simulink model "Modulated TDPC Q4"  (R2021b)
settings: Solver=ode4  StartTime=0.0  StopTime=20  FixedStep=0.0001  RelTol=1e-3
libraries: slpidlib x2
settings Model: Creator=rmkna  LastModifiedBy=rmkna

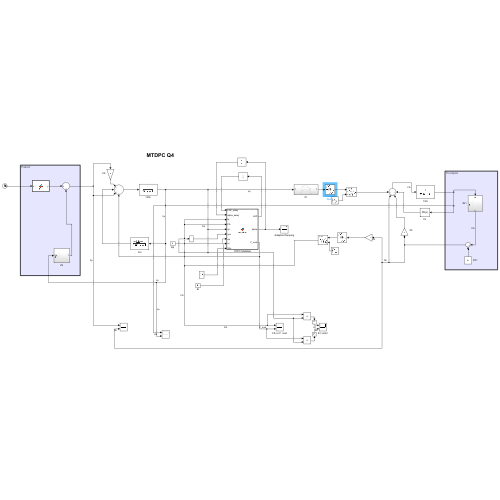
[thumbnail: Simulink's stored preview of the top-level diagram]
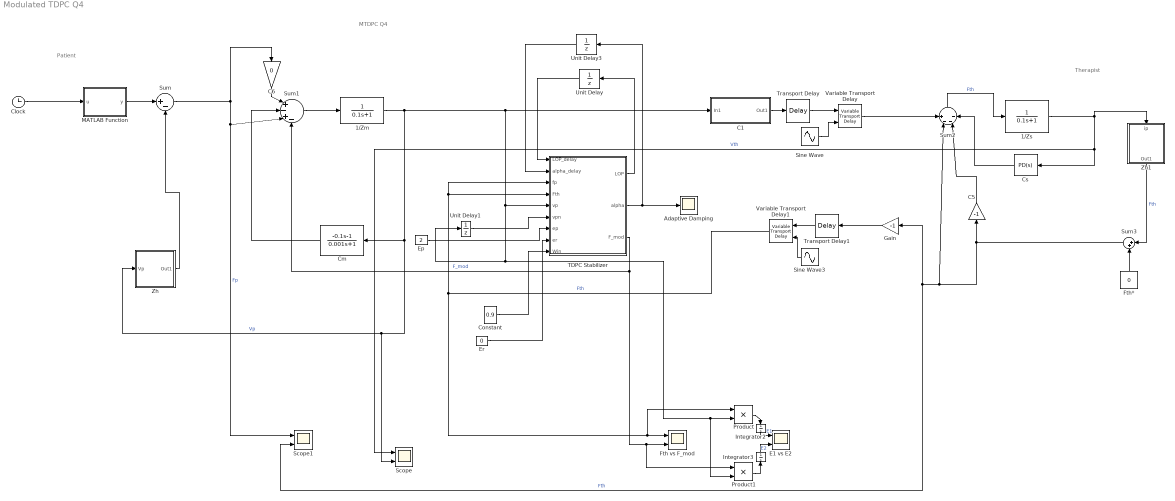
== system Modulated TDPC Q4 ==
  note: MTDPC Q4
  note: Therapist
  note: Patient
  " TDPC Stabilizer" : MATLAB Function  TreatAsAtomicUnit=on
  1/Zm : TransferFcn  Denominator=[0.1 1]
  1/Zs : TransferFcn  Denominator=[0.1 1]
  Adaptive Damping : Scope
  C1 : Subsystem
  "C5 " : Gain  Gain=-1
  "C6 " : Gain  Gain=0
  Clock : Clock
  Cm : TransferFcn  Numerator=[-0.1 -1]  Denominator=[0.001 1]
  Constant : Constant  Value=0.9
  Cs : slpidlib/PID Controller  Controller=PD  Form=Parallel  TimeDomain=Continuous-time  UseExternalTs=off  SampleTime=-1  IntegratorMethod=Forward Euler  FilterMethod=Forward Euler  ControllerParametersSource=internal  P=1000  I=1  D=1  UseFilter=on  N=1000  TunerSelectOption=Transfer Function Based (PID Tuner App)  InitialConditionSource=internal  InitialConditionForIntegrator=0  InitialConditionForFilter=0  DifferentiatorICPrevScaledInput=0  ExternalReset=none  TrackingMode=off  Kt=1  LimitOutput=off  SatLimitsSource=internal  UpperSaturationLimit=inf  LowerSaturationLimit=-inf  LinearizeAsGain=on  AntiWindupMode=none  Kb=1  POutMin=[]  POutMax=[]  IOutMin=[]  IOutMax=[]  DOutMin=[]  DOutMax=[]  NOutMin=[]  NOutMax=[]  SumOutMin=[]  SumOutMax=[]  SaturationOutMin=[]  SaturationOutMax=[]  PParamMin=[]  PParamMax=[]  IParamMin=[]  IParamMax=[]  DParamMin=[]  DParamMax=[]  NParamMin=[]  NParamMax=[]  KbParamMin=[]  KbParamMax=[]  KtParamMin=[]  KtParamMax=[]  KbOutMin=[]  KbOutMax=[]  KtOutMin=[]  KtOutMax=[]  IntegratorOutMin=[]  IntegratorOutMax=[]  FilterOutMin=[]  FilterOutMax=[]  SumI1OutMin=[]  SumI1OutMax=[]  SumI2OutMin=[]  SumI2OutMax=[]  SumI3OutMin=[]  SumI3OutMax=[]  SumI4OutMin=[]  SumI4OutMax=[]  SumDOutMin=[]  SumDOutMax=[]  DifferentiatorOutMin=[]  DifferentiatorOutMax=[]  FilterDiffOutCoefMin=[]  FilterDiffOutCoefMax=[]  ReciprocalOutMin=[]  ReciprocalOutMax=[]  SumDenOutMin=[]  SumDenOutMax=[]  SumNumOutMin=[]  SumNumOutMax=[]  DivideOutMin=[]  DivideOutMax=[]  UdiffTsProdOutMin=[]  UdiffTsProdOutMax=[]  NTsProdOutMin=[]  NTsProdOutMax=[]  UintegralTsProdOutMin=[]  UintegralTsProdOutMax=[]  UngainTsProdOutMin=[]  UngainTsProdOutMax=[]  IntegratorContinuousStateAttributes=''  IntegratorStateMustResolveToSignalObject=off  IntegratorRTWStateStorageClass=Auto  FilterContinuousStateAttributes=''  FilterStateMustResolveToSignalObject=off  FilterRTWStateStorageClass=Auto  ParallelPVariant=InternalParameters  IdealPVariant=Disabled  IVariant=Disabled  DVariant=InternalParameters  IntegratorVariant=Disabled  SatVariant=Disabled  AWVariant=Disabled  PCopyVariant=Disabled  TRVariant=Disabled  FdbkBlocksVariant=Forward  IdealPFdbkVariant=Disabled  SatFdbkVariant=Disabled  DerivativeFilterVariant=ContFilter  NVariant=InternalParameters  NCopyVariant=Disabled  FilterICVariant=InternalICsFilter  IntegratorICVariant=Disabled  ExternalResetVariant=Disabled  TRSumVariant=Passthrough  SumFdbkVariant=Disabled  SumVariant=Sum_PD  TsampFilterVariant=InternalTs  TsampNgainVariant=Passthrough  TsampIntegralVariant=Disabled_SignalSpec  ExternalSaturationOutDataTypeStr=Inherit: Same as second input
  E1 vs E2 : Scope  NumInputPorts=2
  Ep : Constant  Value=2
  Er : Constant  Value=0
  Fth vs F_mod : Scope  NumInputPorts=2
  Fth* : Constant  Value=0  OutDataTypeStr=Inherit: Inherit via back propagation
  Gain : Gain  Gain=-1
  Integrator2 : Integrator
  Integrator3 : Integrator
  MATLAB Function : MATLAB Function  TreatAsAtomicUnit=on
  Product : Product
  Product1 : Product
  Scope : Scope  NumInputPorts=2
  Scope1 : Scope  NumInputPorts=2
  Sine Wave : Sin  Amplitude=0.02  Frequency=12  Phase=pi/2  SampleTime=0
  Sine Wave3 : Sin  Amplitude=0.02  Frequency=12  Phase=pi/2  SampleTime=0
  Sum : Sum  Inputs=|+-
  Sum1 : Sum  Inputs=|+-+-
  Sum2 : Sum  Inputs=+---
  Sum3 : Sum  Inputs=|++
  Transport Delay : TransportDelay  DelayTime=0.1  PadeOrder=3
  Transport Delay1 : TransportDelay  DelayTime=0.1  PadeOrder=3
  Unit Delay : UnitDelay  SampleTime=-1  HasFrameUpgradeWarning=on
  Unit Delay1 : UnitDelay  SampleTime=-1  HasFrameUpgradeWarning=on
  Unit Delay3 : UnitDelay  SampleTime=-1  HasFrameUpgradeWarning=on
  Variable Transport Delay : VariableTransportDelay  PadeOrder=3
  Variable Transport Delay1 : VariableTransportDelay  PadeOrder=3
  Zh : Subsystem
  Zh1 : Subsystem
  wires:
  MATLAB Function/1(y) -> Sum/1
  Sine Wave3/1 -> Variable Transport Delay1/2
  Sum1/1 -> 1/Zm/1
  Transport Delay1/1 -> Variable Transport Delay1/1
  1/Zm/1 -> Scope/2, Zh/1(Vp), Cm/1, Product1/2, Product/2, Unit Delay1/1, " TDPC Stabilizer"/5(vp), C1/1(In1)  "Vp"
  Sine Wave/1 -> Variable Transport Delay/2
  Integrator2/1 -> E1 vs E2/1  "E1"
  Sum3/1 -> Scope1/2, Gain/1, Sum2/2, "C5 "/1  "Fth"
  Integrator3/1 -> E1 vs E2/2  "E2"
  Product1/1 -> Integrator3/1
  Product/1 -> Integrator2/1
  1/Zs/1 -> Zh1/1(ip), Cs/1, Scope/1  "Vth"
  Variable Transport Delay/1 -> Sum2/1
  Unit Delay3/1 -> " TDPC Stabilizer"/2(alpha_delay)
  Er/1 -> " TDPC Stabilizer"/8(er)
  Unit Delay1/1 -> " TDPC Stabilizer"/6(vpn)
  " TDPC Stabilizer"/1(LOP) -> Unit Delay/1
  " TDPC Stabilizer"/3(F_mod) -> Product1/1, Fth vs F_mod/2, Sum1/4  "F_mod"
  C1/1(Out1) -> Transport Delay/1
  Variable Transport Delay1/1 -> Product/1, Fth vs F_mod/1, " TDPC Stabilizer"/3(fp), " TDPC Stabilizer"/4(Fth)  "Fth"
  " TDPC Stabilizer"/2(alpha) -> Adaptive Damping/1, Unit Delay3/1
  Sum/1 -> Scope1/1, Sum1/3, "C6 "/1  "Fp"
  "C5 "/1 -> Sum2/3
  Cm/1 -> Sum1/2
  Transport Delay/1 -> Variable Transport Delay/1
  Unit Delay/1 -> " TDPC Stabilizer"/1(LOP_delay)
  Ep/1 -> " TDPC Stabilizer"/7(ep)
  Sum2/1 -> 1/Zs/1  "Fth"
  Fth*/1 -> Sum3/2
  "C6 "/1 -> Sum1/1
  Zh1/1(Out1) -> Sum3/1  "Fth"
  Clock/1 -> MATLAB Function/1(u)
  Zh/1(Out1) -> Sum/2
  Gain/1 -> Transport Delay1/1
  Cs/1 -> Sum2/4
  Constant/1 -> " TDPC Stabilizer"/9(Win)

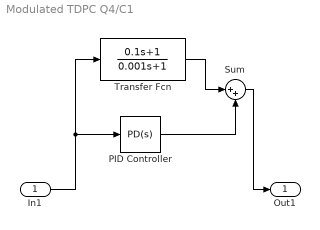
== system Modulated TDPC Q4/C1 ==
  In1 : Inport
  PID Controller : slpidlib/PID Controller  Controller=PD  Form=Parallel  TimeDomain=Continuous-time  UseExternalTs=off  SampleTime=-1  IntegratorMethod=Forward Euler  FilterMethod=Forward Euler  ControllerParametersSource=internal  P=1000  I=1  D=1  UseFilter=on  N=1000  TunerSelectOption=Transfer Function Based (PID Tuner App)  InitialConditionSource=internal  InitialConditionForIntegrator=0  InitialConditionForFilter=0  DifferentiatorICPrevScaledInput=0  ExternalReset=none  TrackingMode=off  Kt=1  LimitOutput=off  SatLimitsSource=internal  UpperSaturationLimit=inf  LowerSaturationLimit=-inf  LinearizeAsGain=on  AntiWindupMode=none  Kb=1  POutMin=[]  POutMax=[]  IOutMin=[]  IOutMax=[]  DOutMin=[]  DOutMax=[]  NOutMin=[]  NOutMax=[]  SumOutMin=[]  SumOutMax=[]  SaturationOutMin=[]  SaturationOutMax=[]  PParamMin=[]  PParamMax=[]  IParamMin=[]  IParamMax=[]  DParamMin=[]  DParamMax=[]  NParamMin=[]  NParamMax=[]  KbParamMin=[]  KbParamMax=[]  KtParamMin=[]  KtParamMax=[]  KbOutMin=[]  KbOutMax=[]  KtOutMin=[]  KtOutMax=[]  IntegratorOutMin=[]  IntegratorOutMax=[]  FilterOutMin=[]  FilterOutMax=[]  SumI1OutMin=[]  SumI1OutMax=[]  SumI2OutMin=[]  SumI2OutMax=[]  SumI3OutMin=[]  SumI3OutMax=[]  SumI4OutMin=[]  SumI4OutMax=[]  SumDOutMin=[]  SumDOutMax=[]  DifferentiatorOutMin=[]  DifferentiatorOutMax=[]  FilterDiffOutCoefMin=[]  FilterDiffOutCoefMax=[]  ReciprocalOutMin=[]  ReciprocalOutMax=[]  SumDenOutMin=[]  SumDenOutMax=[]  SumNumOutMin=[]  SumNumOutMax=[]  DivideOutMin=[]  DivideOutMax=[]  UdiffTsProdOutMin=[]  UdiffTsProdOutMax=[]  NTsProdOutMin=[]  NTsProdOutMax=[]  UintegralTsProdOutMin=[]  UintegralTsProdOutMax=[]  UngainTsProdOutMin=[]  UngainTsProdOutMax=[]  IntegratorContinuousStateAttributes=''  IntegratorStateMustResolveToSignalObject=off  IntegratorRTWStateStorageClass=Auto  FilterContinuousStateAttributes=''  FilterStateMustResolveToSignalObject=off  FilterRTWStateStorageClass=Auto  ParallelPVariant=InternalParameters  IdealPVariant=Disabled  IVariant=Disabled  DVariant=InternalParameters  IntegratorVariant=Disabled  SatVariant=Disabled  AWVariant=Disabled  PCopyVariant=Disabled  TRVariant=Disabled  FdbkBlocksVariant=Forward  IdealPFdbkVariant=Disabled  SatFdbkVariant=Disabled  DerivativeFilterVariant=ContFilter  NVariant=InternalParameters  NCopyVariant=Disabled  FilterICVariant=InternalICsFilter  IntegratorICVariant=Disabled  ExternalResetVariant=Disabled  TRSumVariant=Passthrough  SumFdbkVariant=Disabled  SumVariant=Sum_PD  TsampFilterVariant=InternalTs  TsampNgainVariant=Passthrough  TsampIntegralVariant=Disabled_SignalSpec  ExternalSaturationOutDataTypeStr=Inherit: Same as second input
  Sum : Sum  Inputs=|++
  Transfer Fcn : TransferFcn  Numerator=[0.1 1]  Denominator=[0.001 1]
  Out1 : Outport
  wires:
  In1/1 -> PID Controller/1, Transfer Fcn/1
  Transfer Fcn/1 -> Sum/1
  PID Controller/1 -> Sum/2
  Sum/1 -> Out1/1

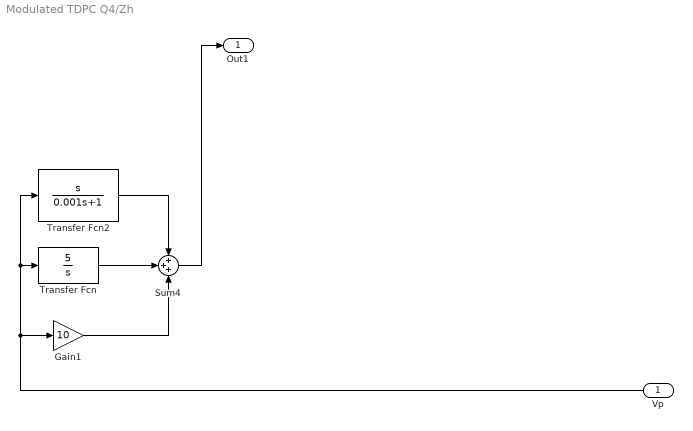
== system Modulated TDPC Q4/Zh ==
  Vp : Inport
  Gain1 : Gain  Gain=10
  Sum4 : Sum  Inputs=3
  Transfer Fcn : TransferFcn  Numerator=[5]  Denominator=[1 0]
  Transfer Fcn2 : TransferFcn  Numerator=[1 0]  Denominator=[0.001 1]
  Out1 : Outport
  wires:
  Vp/1 -> Gain1/1, Transfer Fcn/1, Transfer Fcn2/1
  Sum4/1 -> Out1/1
  Transfer Fcn/1 -> Sum4/2
  Transfer Fcn2/1 -> Sum4/1
  Gain1/1 -> Sum4/3

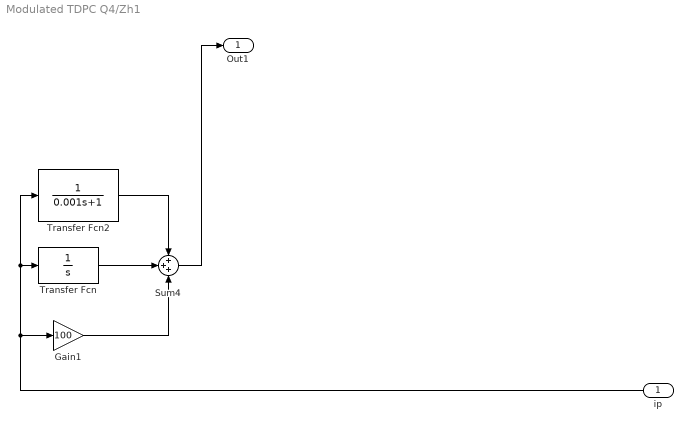
== system Modulated TDPC Q4/Zh1 ==
  ip : Inport
  Gain1 : Gain  Gain=100
  Sum4 : Sum  Inputs=3
  Transfer Fcn : TransferFcn  Denominator=[1 0]
  Transfer Fcn2 : TransferFcn  Denominator=[0.001 1]
  Out1 : Outport
  wires:
  Gain1/1 -> Sum4/3
  Transfer Fcn2/1 -> Sum4/1
  Transfer Fcn/1 -> Sum4/2
  Sum4/1 -> Out1/1
  ip/1 -> Transfer Fcn2/1, Transfer Fcn/1, Gain1/1

== matlab function Modulated TDPC Q4/ TDPC Stabilizer ==
  data: LOP_delay input; alpha_delay input; LOP output; alpha output; fp input; Fth input; F_mod output; vp input; vpn input; ep input; er input; Win input
function [LOP,alpha, F_mod] = Stabilizer(LOP_delay,alpha_delay,fp,Fth,vp,vpn,ep,er,Win)

PL = ((ep-er)*(vp')*vp)+(fp'*vp);

LOP = Win*LOP_delay+(0.001*(PL+(alpha_delay*(vpn')*vpn*Win)));

if LOP>=0
    alpha = 0;
else 
    alpha=(-LOP)/(0.001*(vp')*vp+0.00001);
end

F_mod= Fth+(alpha*vp)+0.00001;

== matlab function Modulated TDPC Q4/MATLAB Function ==
  data: u input; y output
function y = fcn(u)

y = sin(4*u)+ cos(2*u)+ sin(3*u)+cos(u);
